simulink model "Understanding_Control_Systems_3"  (Simulink 8.9)
settings: Solver=VariableStepAuto  StartTime=0.0  StopTime=400  RelTol=1e-3
PreLoadFcn:
  | Car=Simulink.Variant('vehicleType==1')
  | SportsCar=Simulink.Variant('vehicleType==2')
  | Truck=Simulink.Variant('vehicleType==3')
  | 
  | vehicleType=1
libraries: MeldasLibrary x5, simulink x1
settings Model: Creator=mulusoy  LastModifiedBy=mulusoy
settings DataIOCC: LimitDataPoints=off  SaveFormat=Dataset  SignalLoggingSaveFormat=Dataset
settings OptimizationCC: LifeSpan=auto
settings DebuggingCC: UnderspecifiedInitializationDetection=Simplified  MergeDetectMultiDrivingBlocksExec=error  FcnCallInpInsideContextMsg=error  StateNameClashWarn=none  SFUnexpectedBacktrackingDiag=error  SFNoUnconditionalDefaultTransitionDiag=error  SFExecutionAtInitializationDiag=warning
settings HardwareCC: ProdBitPerPointer=64  ProdBitPerSizeT=64  ProdBitPerPtrDiffT=64  ProdLargestAtomicFloat=Float  ProdIntDivRoundTo=Zero  ProdEndianess=LittleEndian  ProdWordSize=64  ProdHWDeviceType=Intel->x86-64 (Windows64)
settings ModelReferenceCC: PropagateSignalLabelsOutOfModel=on
settings GRTTargetCC: TargetLangStandard=C99 (ISO)  GeneratePreprocessorConditionals=Use local settings  CombineOutputUpdateFcns=on  GRTInterface=off
settings ConfigComp: CovMetricSettings=dswe  CovHtmlReporting=off  CovSaveCumulativeToWorkspaceVar=off  CovSaveSingleToWorkspaceVar=off  CovExternalEMLEnable=on

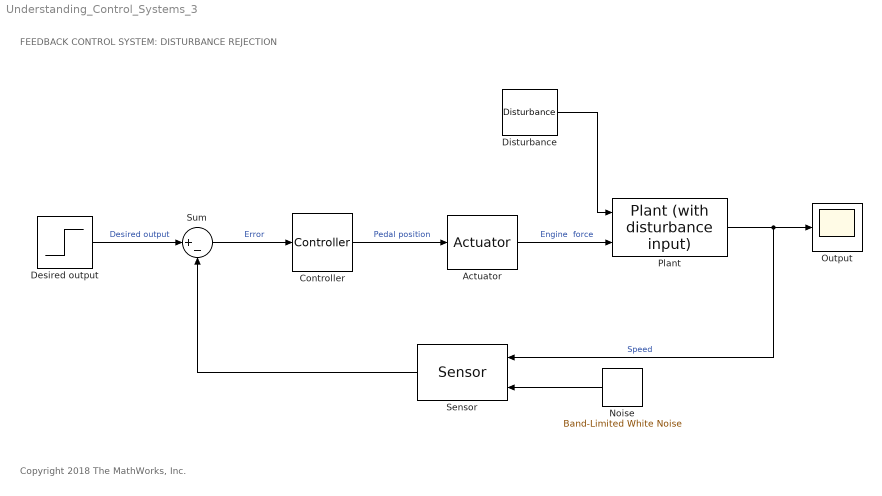
== system Understanding_Control_Systems_3 ==
  note: Copyright 2018 The MathWorks, Inc.
  note: FEEDBACK CONTROL SYSTEM: DISTURBANCE REJECTION
  Actuator : MeldasLibrary/Actuator  SystemSampleTime=-1
      settings: SourceProductName=Melda's Library
  Controller : MeldasLibrary/Controller  SystemSampleTime=-1
      settings: SourceProductName=Melda's Library
  Desired output : Step  Time=5  After=20  SampleTime=0
  Disturbance : MeldasLibrary/Disturbance  SystemSampleTime=-1
      settings: SourceProductName=Melda's Library
  Noise : simulink/Sources/Band-Limited White Noise  Cov=0.01  Ts=0.1  seed=[23341]
  Output : Scope
  Plant : MeldasLibrary/Plant (with disturbance input)  vehicleType=Car
      settings: SourceProductName=Melda's Library
  Sensor : MeldasLibrary/Sensor  SystemSampleTime=-1
      settings: SourceProductName=Melda's Library
  Sum : Sum  Inputs=|+-
  wires:
  Controller/1 -> Actuator/1  "Pedal position"
  Actuator/1 -> Plant/2  "Engine  force"
  Plant/1 -> Sensor/1, Output/1  "Speed"
  Disturbance/1 -> Plant/1
  Noise/1 -> Sensor/2
  Desired output/1 -> Sum/1  "Desired output"
  Sensor/1 -> Sum/2
  Sum/1 -> Controller/1  "Error"
